simulink model "SimulationWithMotor"  (R2023a)
settings: configuration reference "SharedConfig" (kept outside this file)
undefined symbols (not defined in the file): Analyse, check, config_motor, k_FW, motormap, motormap2
settings Model: PauseTimes=35  Creator=maximilian.tschochne  LastModifiedBy=ge49hus
settings ConfigSetRef: SourceName=SharedConfig  SourceLocation=Base Workspace

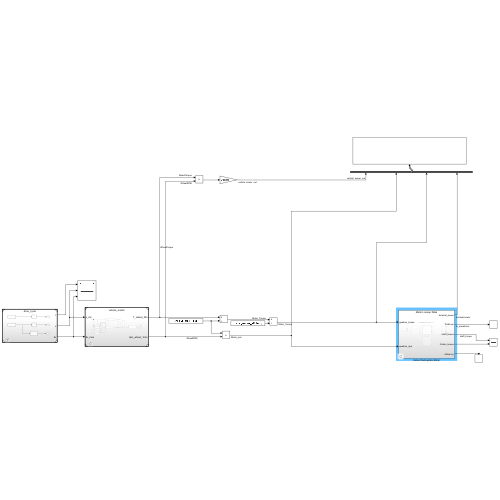
[thumbnail: Simulink's stored preview of the top-level diagram]
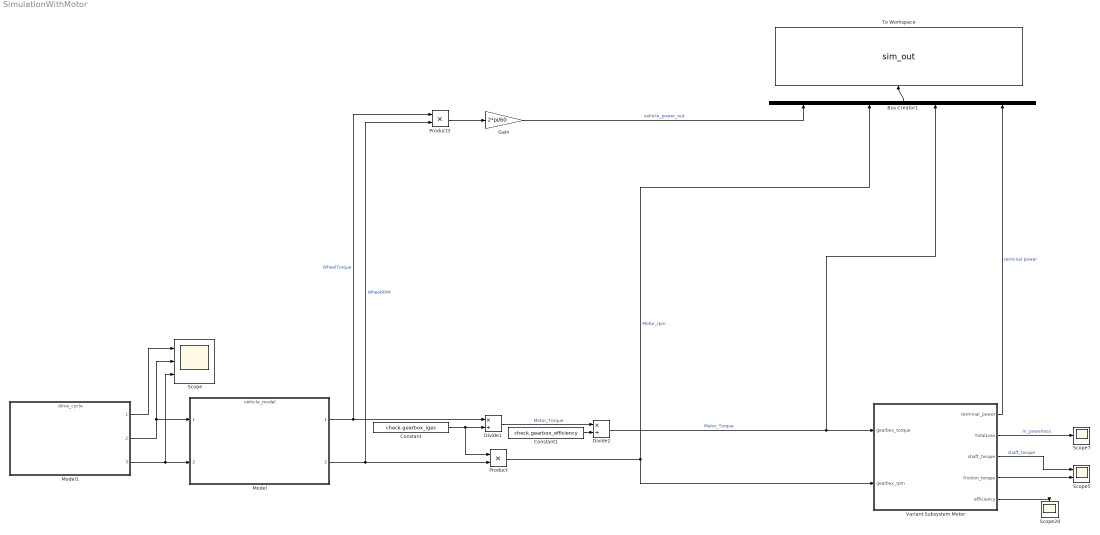
== system SimulationWithMotor ==
  Bus Creator1 : BusCreator  Inputs=4
  Constant : Constant  Value=check.gearbox_iges
  Constant1 : Constant  Value=check.gearbox_efficiency
  Divide1 : Product  Inputs=*/
  Divide2 : Product  Inputs=*/
  Gain : Gain  Gain=2*pi/60
  Model : ModelReference  ModelNameDialog=vehicle_model.slx  SimulationMode=Normal  ModelReferenceVersion=2.0
  Model1 : ModelReference  ModelNameDialog=drive_cycle.slx  SimulationMode=Normal  ModelReferenceVersion=1.0
  Product : Product
  Product3 : Product
  Scope : Scope  NumInputPorts=3
  Scope20 : Scope
  Scope5 : Scope  NumInputPorts=2
  Scope7 : Scope
  To Workspace : ToWorkspace  VariableName=sim_out  SaveFormat=Timeseries  SampleTime=-1
  Variant Subsystem Motor : Subsystem  Variant=on
  wires:
  Model1/1 -> Scope/1
  Model1/2 -> Scope/2, Model/1
  Model1/3 -> Scope/3, Model/2
  Bus Creator1/1 -> To Workspace/1
  Gain/1 -> Bus Creator1/1  "vehicle_power_out"
  Model/1 -> Product3/1, Divide1/1  "WheelTorque"
  Product3/1 -> Gain/1
  Variant Subsystem Motor/2(TotalLoss) -> Scope7/1  "m_powerloss"
  Variant Subsystem Motor/3(shaft_torque) -> Scope5/1  "shaft_torque"
  Variant Subsystem Motor/5(efficiency) -> Scope20/1
  Variant Subsystem Motor/4(friction_torque) -> Scope5/2
  Model/2 -> Product/2, Product3/2  "WheelRPM"
  Divide1/1 -> Divide2/1  "Motor_Torque"
  Constant/1 -> Product/1, Divide1/2
  Constant1/1 -> Divide2/2
  Product/1 -> Variant Subsystem Motor/2(gearbox_rpm), Bus Creator1/2  "Motor_rpm"
  Divide2/1 -> Bus Creator1/3, Variant Subsystem Motor/1(gearbox_torque)  "Motor_Torque"
  Variant Subsystem Motor/1(terminal_power) -> Bus Creator1/4  "terminal power"

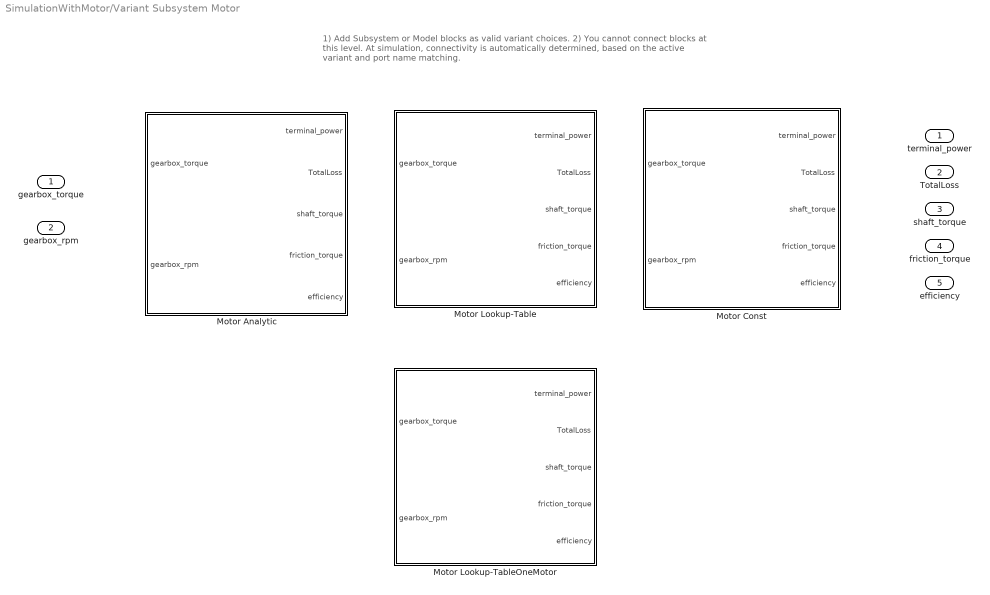
== system SimulationWithMotor/Variant Subsystem Motor ==
  note: 1) Add Subsystem or Model blocks as valid variant choices.
      | 2) You cannot connect blocks at this level. At simulation, connectivity is automatically
      | determined, based on the active variant and port name matching.
  gearbox_torque : Inport
  gearbox_rpm : Inport  Port=2
  Motor Analytic : Subsystem  VariantControl="Motor_Mode == \"Analytic\""
  Motor Const : Subsystem  VariantControl="Motor_Mode == \"Const\""
  Motor Lookup-Table : Subsystem  VariantControl="Motor_Mode == \"Lookup\""
  Motor Lookup-TableOneMotor : Subsystem  VariantControl="Motor_Mode == \"LookupOneMotor\""
  terminal_power : Outport
  TotalLoss : Outport  Port=2
  shaft_torque : Outport  Port=3
  friction_torque : Outport  Port=4
  efficiency : Outport  Port=5

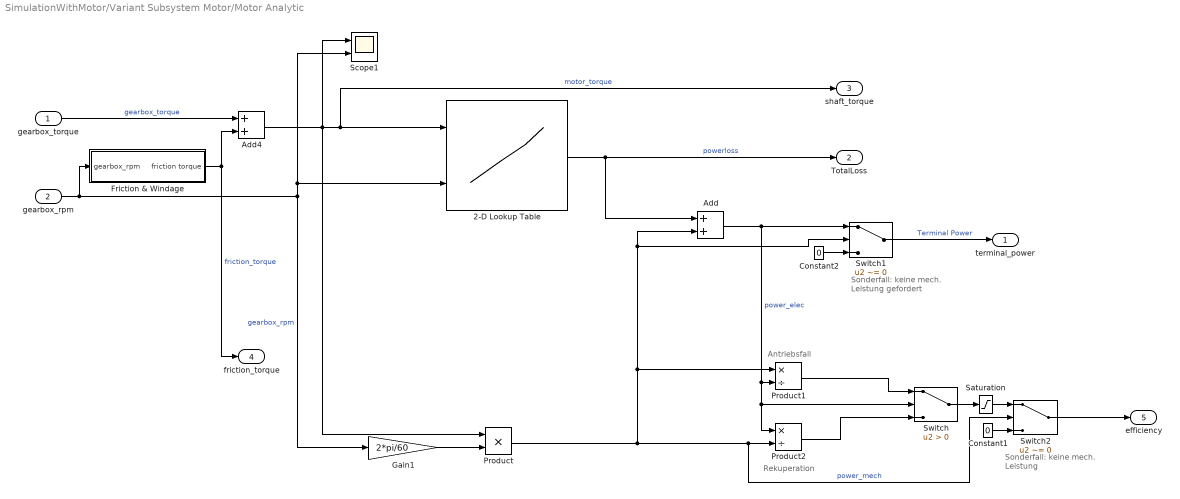
== system SimulationWithMotor/Variant Subsystem Motor/Motor Analytic ==
  note: Sonderfall:
      | keine mech. Leistung
  note: Antriebsfall
  note: Rekuperation
  note: Sonderfall: keine mech.
      | Leistung gefordert
  gearbox_torque : Inport
  gearbox_rpm : Inport  Port=2
  2-D Lookup Table : Lookup_n-D  BreakpointsForDimension1=Analyse.Betriebsdaten.M_vec(end:-1:1)  BreakpointsForDimension2=Analyse.Betriebsdaten.n_m_mesh(Analyse.Optionen.M_tics,:)  Table=Analyse.Verluste.P_vges_mesh(end:-1:1,:)  InternalRulePriority=Speed  RndMeth=Simplest
      settings: InputPortMap=u0,u1
  Add : Sum
  Add4 : Sum
  Constant1 : Constant  Value=0
  Constant2 : Constant  Value=0
  Friction & Windage : Subsystem
  Gain1 : Gain  Gain=2*pi/60
  Product : Product
  Product1 : Product  Inputs=*/
  Product2 : Product  Inputs=*/
  Saturation : Saturate  UpperLimit=inf  LowerLimit=0
  Scope1 : Scope  NumInputPorts=2
  Switch : Switch  Criteria=u2 > Threshold  SaturateOnIntegerOverflow=off  InputSameDT=off
  Switch1 : Switch  Criteria=u2 ~= 0  SaturateOnIntegerOverflow=off  InputSameDT=off
  Switch2 : Switch  Criteria=u2 ~= 0  SaturateOnIntegerOverflow=off  InputSameDT=off
  terminal_power : Outport
  TotalLoss : Outport  Port=2
  shaft_torque : Outport  Port=3
  friction_torque : Outport  Port=4
  efficiency : Outport  Port=5
  wires:
  gearbox_rpm/1 -> Friction & Windage/1(gearbox_rpm), Scope1/2, 2-D Lookup Table/2, Gain1/1  "gearbox_rpm"
  2-D Lookup Table/1 -> Add/1, TotalLoss/1  "powerloss"
  Product/1 -> Switch2/2, Product2/2, Switch1/2, Add/2, Product1/1  "power_mech"
  Add/1 -> Switch1/1, Product2/1, Switch/2, Product1/2  "power_elec"
  Product2/1 -> Switch/3
  Add4/1 -> Scope1/1, Product/1, shaft_torque/1, 2-D Lookup Table/1  "motor_torque"
  Switch2/1 -> efficiency/1
  Gain1/1 -> Product/2
  Constant2/1 -> Switch1/3
  Switch1/1 -> terminal_power/1  "Terminal Power"
  Product1/1 -> Switch/1
  gearbox_torque/1 -> Add4/1  "gearbox_torque"
  Friction & Windage/1(friction torque) -> friction_torque/1, Add4/2  "friction_torque"
  Switch/1 -> Saturation/1
  Constant1/1 -> Switch2/3
  Saturation/1 -> Switch2/1

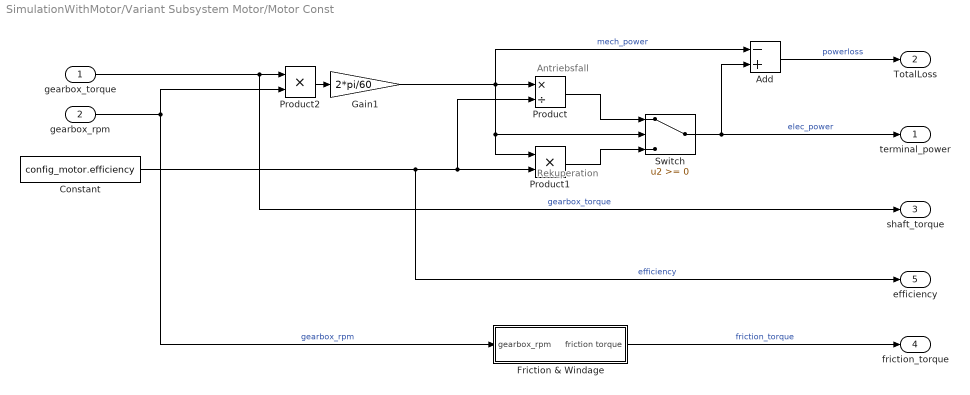
== system SimulationWithMotor/Variant Subsystem Motor/Motor Const ==
  note: Rekuperation
  note: Antriebsfall
  gearbox_torque : Inport
  gearbox_rpm : Inport  Port=2
  Add : Sum  Inputs=-+
  Constant : Constant  Value=config_motor.efficiency
  Friction & Windage : Subsystem
  Gain1 : Gain  Gain=2*pi/60
  Product : Product  Inputs=*/
  Product1 : Product  Inputs=**
  Product2 : Product
  Switch : Switch  SaturateOnIntegerOverflow=off  InputSameDT=off
  terminal_power : Outport
  TotalLoss : Outport  Port=2
  shaft_torque : Outport  Port=3
  friction_torque : Outport  Port=4
  efficiency : Outport  Port=5
  wires:
  Product2/1 -> Gain1/1
  Constant/1 -> efficiency/1, Product1/2, Product/2  "efficiency"
  Product/1 -> Switch/1
  Product1/1 -> Switch/3
  Add/1 -> TotalLoss/1  "powerloss"
  Switch/1 -> terminal_power/1, Add/2  "elec_power"
  gearbox_rpm/1 -> Friction & Windage/1(gearbox_rpm), Product2/2  "gearbox_rpm"
  Gain1/1 -> Add/1, Product1/1, Switch/2, Product/1  "mech_power"
  gearbox_torque/1 -> Product2/1, shaft_torque/1  "gearbox_torque"
  Friction & Windage/1(friction torque) -> friction_torque/1  "friction_torque"

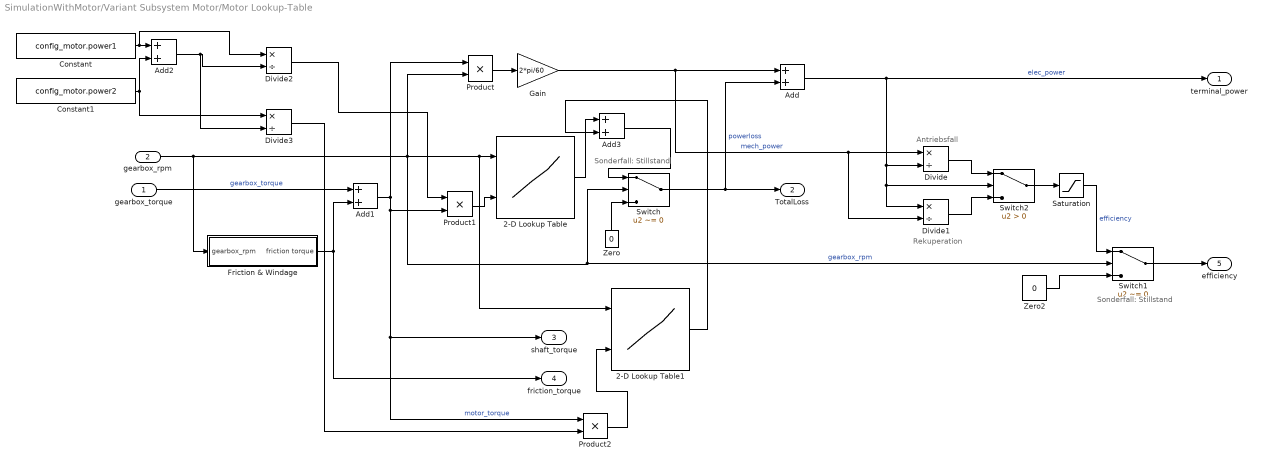
== system SimulationWithMotor/Variant Subsystem Motor/Motor Lookup-Table ==
  note: Sonderfall: Stillstand
  note: Rekuperation
  note: Antriebsfall
  note: Sonderfall: Stillstand
  gearbox_torque : Inport
  gearbox_rpm : Inport  Port=2
  2-D Lookup Table : Lookup_n-D  BreakpointsForDimension1=motormap.nVec  BreakpointsForDimension2=motormap.MVec  Table=motormap.Loss  InternalRulePriority=Speed  RndMeth=Simplest
      settings: InputPortMap=u0,u1
  2-D Lookup Table1 : Lookup_n-D  BreakpointsForDimension1=motormap2.nVec  BreakpointsForDimension2=motormap2.MVec  Table=motormap2.Loss  InternalRulePriority=Speed  RndMeth=Simplest
      settings: InputPortMap=u0,u1
  Add{,1..3} (4 alike) : Sum
  Constant : Constant  Value=config_motor.power1
  Constant1 : Constant  Value=config_motor.power2
  Divide{,1..3} (4 alike) : Product  Inputs=*/
  Friction & Windage : Subsystem
  Gain : Gain  Gain=2*pi/60
  Product : Product
  Product1 : Product
  Product2 : Product
  Saturation : Saturate  UpperLimit=inf  LowerLimit=0
  Switch : Switch  Criteria=u2 ~= 0  Threshold=1  SaturateOnIntegerOverflow=off  InputSameDT=off
  Switch1 : Switch  Criteria=u2 ~= 0  SaturateOnIntegerOverflow=off  InputSameDT=off
  Switch2 : Switch  Criteria=u2 > Threshold  SaturateOnIntegerOverflow=off  InputSameDT=off
  Zero : Constant  Value=0  OutDataTypeStr=Inherit: Inherit via back propagation
  Zero2 : Constant  Value=0  OutDataTypeStr=Inherit: Inherit via back propagation
  terminal_power : Outport
  TotalLoss : Outport  Port=2
  shaft_torque : Outport  Port=3
  friction_torque : Outport  Port=4
  efficiency : Outport  Port=5
  wires:
  gearbox_torque/1 -> Add1/1  "gearbox_torque"
  2-D Lookup Table/1 -> Add3/1
  Product/1 -> Gain/1
  Gain/1 -> Divide/1, Divide1/2, Add/1  "mech_power"
  Switch/1 -> TotalLoss/1, Add/2  "powerloss"
  Zero/1 -> Switch/3
  Add/1 -> Switch2/2, Divide1/1, Divide/2, terminal_power/1  "elec_power"
  Switch1/1 -> efficiency/1
  Zero2/1 -> Switch1/3
  Switch2/1 -> Saturation/1
  Divide/1 -> Switch2/1
  Divide1/1 -> Switch2/3
  Saturation/1 -> Switch1/1  "efficiency"
  gearbox_rpm/1 -> 2-D Lookup Table1/1, 2-D Lookup Table/1, Switch1/2, Switch/2, Product/2, Friction & Windage/1(gearbox_rpm)  "gearbox_rpm"
  Add1/1 -> Product1/2, Product2/1, shaft_torque/1, Product/1  "motor_torque"
  Friction & Windage/1(friction torque) -> Add1/2, friction_torque/1
  Constant/1 -> Divide2/1, Add2/1
  Constant1/1 -> Add2/2, Divide3/1
  Add2/1 -> Divide3/2, Divide2/2
  Divide2/1 -> Product1/1
  Product1/1 -> 2-D Lookup Table/2
  Product2/1 -> 2-D Lookup Table1/2
  Divide3/1 -> Product2/2
  2-D Lookup Table1/1 -> Add3/2
  Add3/1 -> Switch/1

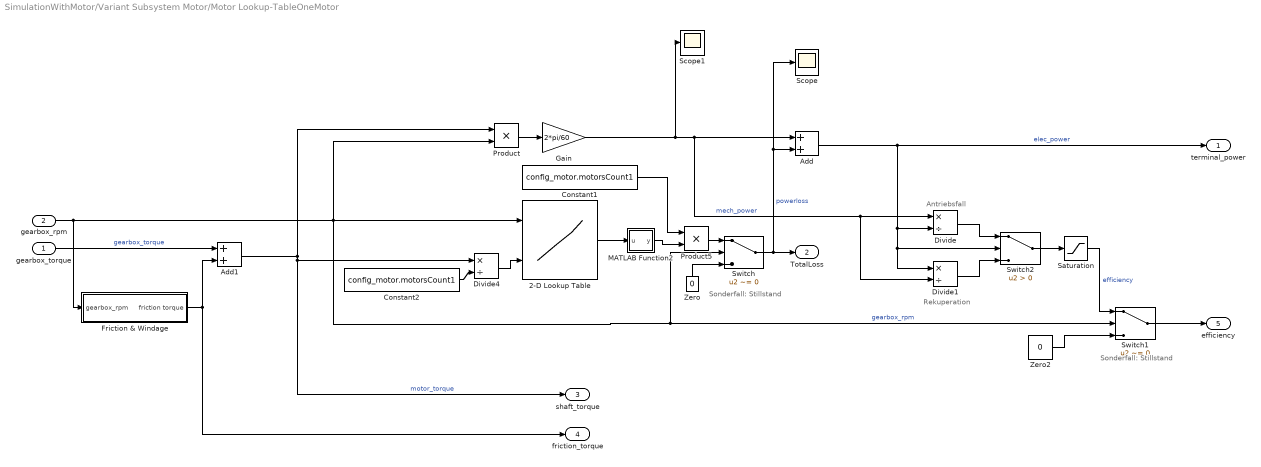
== system SimulationWithMotor/Variant Subsystem Motor/Motor Lookup-TableOneMotor ==
  note: Sonderfall: Stillstand
  note: Rekuperation
  note: Antriebsfall
  note: Sonderfall: Stillstand
  gearbox_torque : Inport
  gearbox_rpm : Inport  Port=2
  2-D Lookup Table : Lookup_n-D  BreakpointsForDimension1=motormap.nVec  BreakpointsForDimension2=motormap.MVec  Table=motormap.Loss  InternalRulePriority=Speed  RndMeth=Simplest
      settings: InputPortMap=u0,u1
  Add : Sum
  Add1 : Sum
  Constant1 : Constant  Value=config_motor.motorsCount1
  Constant2 : Constant  Value=config_motor.motorsCount1
  Divide : Product  Inputs=*/
  Divide1 : Product  Inputs=*/
  Divide4 : Product  Inputs=*/
  Friction & Windage : Subsystem
  Gain : Gain  Gain=2*pi/60
  MATLAB Function2 : MATLAB Function  TreatAsAtomicUnit=on
  Product : Product
  Product5 : Product
  Saturation : Saturate  UpperLimit=inf  LowerLimit=0
  Scope : Scope
  Scope1 : Scope
  Switch : Switch  Criteria=u2 ~= 0  Threshold=1  SaturateOnIntegerOverflow=off  InputSameDT=off
  Switch1 : Switch  Criteria=u2 ~= 0  SaturateOnIntegerOverflow=off  InputSameDT=off
  Switch2 : Switch  Criteria=u2 > Threshold  SaturateOnIntegerOverflow=off  InputSameDT=off
  Zero : Constant  Value=0  OutDataTypeStr=Inherit: Inherit via back propagation
  Zero2 : Constant  Value=0  OutDataTypeStr=Inherit: Inherit via back propagation
  terminal_power : Outport
  TotalLoss : Outport  Port=2
  shaft_torque : Outport  Port=3
  friction_torque : Outport  Port=4
  efficiency : Outport  Port=5
  wires:
  gearbox_torque/1 -> Add1/1  "gearbox_torque"
  Product/1 -> Gain/1
  Gain/1 -> Scope1/1, Divide/1, Divide1/2, Add/1  "mech_power"
  Switch/1 -> Add/2, Scope/1, TotalLoss/1  "powerloss"
  Zero/1 -> Switch/3
  Add/1 -> Switch2/2, Divide1/1, Divide/2, terminal_power/1  "elec_power"
  Switch1/1 -> efficiency/1
  Zero2/1 -> Switch1/3
  Switch2/1 -> Saturation/1
  Divide/1 -> Switch2/1
  Divide1/1 -> Switch2/3
  Saturation/1 -> Switch1/1  "efficiency"
  gearbox_rpm/1 -> 2-D Lookup Table/1, Switch1/2, Switch/2, Product/2, Friction & Windage/1(gearbox_rpm)  "gearbox_rpm"
  Add1/1 -> Divide4/1, shaft_torque/1, Product/1  "motor_torque"
  Friction & Windage/1(friction torque) -> friction_torque/1, Add1/2
  2-D Lookup Table/1 -> MATLAB Function2/1(u)
  MATLAB Function2/1(y) -> Product5/2
  Divide4/1 -> 2-D Lookup Table/2
  Product5/1 -> Switch/1
  Constant2/1 -> Divide4/2
  Constant1/1 -> Product5/1

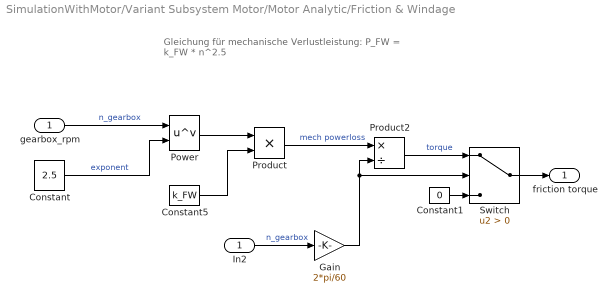
== system SimulationWithMotor/Variant Subsystem Motor/Motor Analytic/Friction & Windage ==
  note: Gleichung für mechanische Verlustleistung:
      | P_FW = k_FW * n^2.5
  gearbox_rpm : Inport
  Constant : Constant  Value=2.5
  Constant1 : Constant  Value=0
  Constant5 : Constant  Value=k_FW
  Gain : Gain  Gain=2*pi/60
  In2 : InportShadow
  Power : Math  Operator=pow
  Product : Product
  Product2 : Product  Inputs=*/
  Switch : Switch  Criteria=u2 > Threshold  SaturateOnIntegerOverflow=off  InputSameDT=off
  friction torque : Outport
  wires:
  gearbox_rpm/1 -> Power/1  "n_gearbox"
  Constant/1 -> Power/2  "exponent"
  Power/1 -> Product/1
  Constant5/1 -> Product/2
  Product/1 -> Product2/1  "mech powerloss"
  Product2/1 -> Switch/1  "torque"
  In2/1 -> Gain/1  "n_gearbox"
  Gain/1 -> Product2/2, Switch/2
  Switch/1 -> friction torque/1
  Constant1/1 -> Switch/3

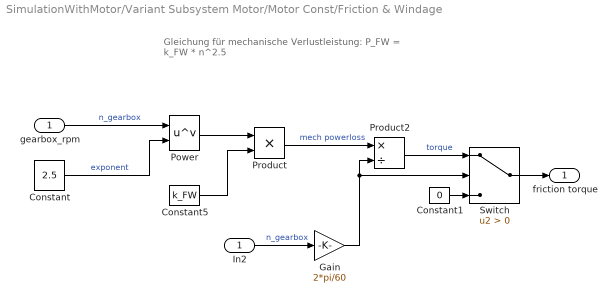
== system SimulationWithMotor/Variant Subsystem Motor/Motor Const/Friction & Windage ==
  note: Gleichung für mechanische Verlustleistung:
      | P_FW = k_FW * n^2.5
  gearbox_rpm : Inport
  Constant : Constant  Value=2.5
  Constant1 : Constant  Value=0
  Constant5 : Constant  Value=k_FW
  Gain : Gain  Gain=2*pi/60
  In2 : InportShadow
  Power : Math  Operator=pow
  Product : Product
  Product2 : Product  Inputs=*/
  Switch : Switch  Criteria=u2 > Threshold  SaturateOnIntegerOverflow=off  InputSameDT=off
  friction torque : Outport
  wires:
  gearbox_rpm/1 -> Power/1  "n_gearbox"
  Constant/1 -> Power/2  "exponent"
  Power/1 -> Product/1
  Constant5/1 -> Product/2
  Product/1 -> Product2/1  "mech powerloss"
  Product2/1 -> Switch/1  "torque"
  In2/1 -> Gain/1  "n_gearbox"
  Gain/1 -> Product2/2, Switch/2
  Switch/1 -> friction torque/1
  Constant1/1 -> Switch/3

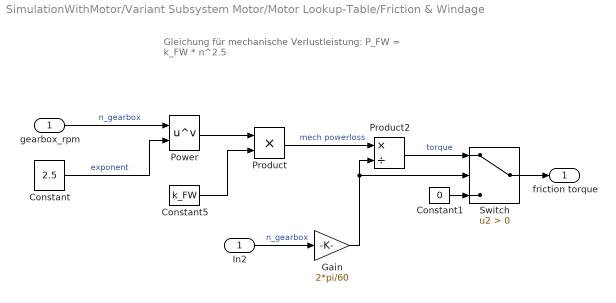
== system SimulationWithMotor/Variant Subsystem Motor/Motor Lookup-Table/Friction & Windage ==
  note: Gleichung für mechanische Verlustleistung:
      | P_FW = k_FW * n^2.5
  gearbox_rpm : Inport
  Constant : Constant  Value=2.5
  Constant1 : Constant  Value=0
  Constant5 : Constant  Value=k_FW
  Gain : Gain  Gain=2*pi/60
  In2 : InportShadow
  Power : Math  Operator=pow
  Product : Product
  Product2 : Product  Inputs=*/
  Switch : Switch  Criteria=u2 > Threshold  SaturateOnIntegerOverflow=off  InputSameDT=off
  friction torque : Outport
  wires:
  gearbox_rpm/1 -> Power/1  "n_gearbox"
  Constant/1 -> Power/2  "exponent"
  Power/1 -> Product/1
  Constant5/1 -> Product/2
  Product/1 -> Product2/1  "mech powerloss"
  Product2/1 -> Switch/1  "torque"
  In2/1 -> Gain/1  "n_gearbox"
  Gain/1 -> Product2/2, Switch/2
  Switch/1 -> friction torque/1
  Constant1/1 -> Switch/3

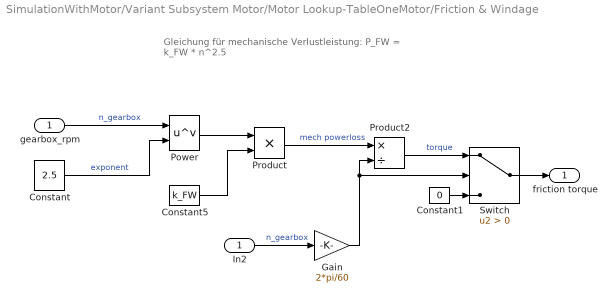
== system SimulationWithMotor/Variant Subsystem Motor/Motor Lookup-TableOneMotor/Friction & Windage ==
  note: Gleichung für mechanische Verlustleistung:
      | P_FW = k_FW * n^2.5
  gearbox_rpm : Inport
  Constant : Constant  Value=2.5
  Constant1 : Constant  Value=0
  Constant5 : Constant  Value=k_FW
  Gain : Gain  Gain=2*pi/60
  In2 : InportShadow
  Power : Math  Operator=pow
  Product : Product
  Product2 : Product  Inputs=*/
  Switch : Switch  Criteria=u2 > Threshold  SaturateOnIntegerOverflow=off  InputSameDT=off
  friction torque : Outport
  wires:
  gearbox_rpm/1 -> Power/1  "n_gearbox"
  Constant/1 -> Power/2  "exponent"
  Power/1 -> Product/1
  Constant5/1 -> Product/2
  Product/1 -> Product2/1  "mech powerloss"
  Product2/1 -> Switch/1  "torque"
  In2/1 -> Gain/1  "n_gearbox"
  Gain/1 -> Product2/2, Switch/2
  Switch/1 -> friction torque/1
  Constant1/1 -> Switch/3

== matlab function SimulationWithMotor/Variant Subsystem Motor/Motor Lookup-TableOneMotor/MATLAB Function2 ==
  data: u input; y output
function y = fcn(u)

if isnan(u)
    %warning('P_motor_111 is NaN. Setting it to 0.');
    y = 0;
else
    y = u;
end
